simulink model "sine"  (R2019b)
settings: Solver=VariableStepAuto  StartTime=0.0  StopTime=3000  RelTol=1e-3
undefined symbols (not defined in the file): xc7vx485tffg1157
libraries: ModelComposer x2
settings Model: Creator=abehbood  LastModifiedBy=abehbood

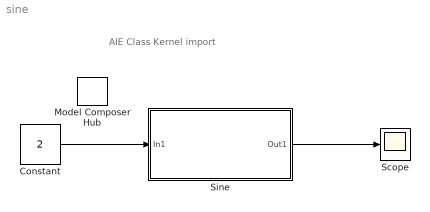
== system sine ==
  note: AIE Class Kernel import
  Constant : Constant  Value=2  VectorParams1D=off  OutDataTypeStr=int16  SampleTime=1
  Model Composer Hub : ModelComposer/Model Composer Hub  CodeGeneration=off  SubsystemName=Sine  TargetDirectory=./code  ExportType=AI Engines  IpVendor=xilinx.com  IpLibrary=hls  IpVersion=1.0  IpHWLanguage=Verilog  AieCompilerOptions={}  CreateTestbench=on  TestbenchStackSize=10  RunAieSim=on  AieSimTimeout=50000  LaunchVitisAnalyzer=off  RunX86Sim=off  X86SimTimeout=10  ProjDevice=xc7vx485tffg1157-1  ProjDevicePart=xc7vx485tffg1157-1  SamplePeriod=-1  ClockFrequency=200  DataPathParallelism=1
  Scope : Scope
  Sine : Subsystem
  wires:
  Constant/1 -> Sine/1(In1)
  Sine/1(Out1) -> Scope/1

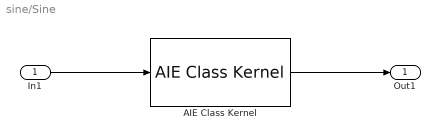
== system sine/Sine ==
  In1 : Inport
  AIE Class Kernel : ModelComposer/AIE Class Kernel  KernelAllAttrs=s[12;12;9;9;19;14;21;23;24;21;12;24;26;26;26;27;28;9;21;23;23;23;24;25;14;19;19;29]@FunctionNameDeclFileNamePortNamesPortTypesPortSerializedTypesPortDirectionsPortWindowSizeEnablesPortWindowMarginEnablesPortSynchronicityEnablesPortSignalSizeEnablesFunctionDeclFunctionTemplateSpecKindFunctionTemplateParamNamesFunctionTemplateParamKindsFunctionTemplateParamTypesFunctionTemplateParamValuesFunctionTemplateParamEnablesClassDeclClassTemplateSpecKindClassTemplateParamNamesClassTemplateParamKindsClassTemplateParamTypesClassTemplateParamValuesClassTemplateParamEnablesClassCtorDeclsClassCtorParamNamesClassCtorParamTypesClassCtorParamSerializedTypes[1 1]@C[28 1]@t8@generatet16@../../src/sine.hC[2 1]@t5@scalet3@outC[2 1]@t5@int16t22@output_window_cint16 *C[2 1]@t6@{Bi16}t34@{P{Toutput_window{1{t{Scint16}}}}}C[2 1]@t5@inputt6@outputC[2 1]@l0@l1@C[2 1]@l0@l0@C[2 1]@l1@l1@C[2 1]@l0@l0@t54@void generate(int16 scale, output_window_cint16 * out)t4@nonee[0 1]@e[0 1]@e[0 1]@e[0 1]@e[0 1]@t14@class SineGen;t4@nonee[0 1]@e[0 1]@e[0 1]@e[0 1]@e[0 1]@e[0 1]@e[0 1]@e[0 1]@e[0 1]@  PortNames={'scale'; 'out'}  PortSerializedTypes={'{Bi16}'; '{P{Toutput_window{1{t{Scint16}}}}}'}  PortWindowSizes={0.000000000000000000e+00; 1.600000000000000000e+01}  PortWindowMargins={0.000000000000000000e+00; 0.000000000000000000e+00}  PortSynchronicities={'auto'; 'auto'}  PortSignalSizes={0.000000000000000000e+00; 0.000000000000000000e+00}  ClassTemplateSpecKind=none  ClassTemplateParamNames={}  ClassTemplateParamKinds={}  ClassTemplateParamTypes={}  ClassTemplateParamValues={}  ClassCtorParamNames={}  ClassCtorParamSerializedTypes={}  ClassCtorParamValues={}  ClassIndex=1  ClassCtorIndex=0  ClassTabVisible=on  ClassTemplateParamsVisible=off  ClassCtorDeclVisible=off  ClassCtorParamsVisible=off  FunctionTabVisible=on  PortAttrs={ 'input', 'scale', 'int16', '', '', 'auto', ''; 'output', 'out', 'output_window_cint16 *', '16', '', 'auto', '' }  PortAttrsEnables={'off', 'off', 'off', 'off', 'off', 'on', 'off';'off', 'off', 'off', 'on', 'off', 'on', 'off'}  ClassDeclTypeOptions=C[1 1]@t14@class SineGen;  ClassDecl=class SineGen;  ClassTemplateParams={}  ClassTemplateParamsEnables={}  ClassCtorDeclTypeOptions=C[1 1]@t7@<empty>  ClassCtorDecl=<empty>  ClassCtorParams={}  KernelHeaderFile=src/sine.h  KernelClassName=SineGen  KernelFunction=generate  KernelSourceFile=src/sine.cpp  KernelSearchPaths={}  PreProcOptions={}  CoreRuntimeRatio=0.9  KernelLocSpec=off  ColRowLocation=[0 0]
  Out1 : Outport
  wires:
  In1/1 -> AIE Class Kernel/1
  AIE Class Kernel/1 -> Out1/1
